simulink model "pendulum_sim"  (Simulink 7.7)
settings: Solver=ode45  StartTime=0.0  StopTime=100  RelTol=1e-3
values from neighbouring files (symbols this model uses):
  kd_th = -2*zeta_th*wn_th*AP.m2*AP.ell    [param.m]
  kd_z = AP.m2/AP.m1/AP.g*(-AP.b/AP.m2 + 2*zeta_z*wn_z)    [param.m]
  kp_th = -AP.F_max/A_th    [param.m]
  kp_z = A_th/A_z    (= 0.0174532925199)    [param.m]
undefined symbols (not defined in the file or in its folder): drawPendulum
settings Model: Creator=beard  LastModifiedBy=beard
settings OptimizationCC: InitFltsAndDblsToZero=on
settings DebuggingCC: StrictBusMsg=Warning

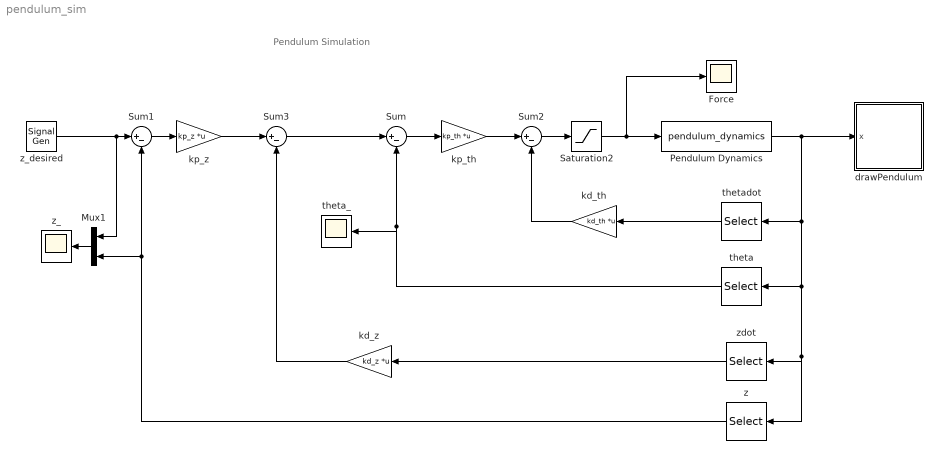
== system pendulum_sim ==
  note: Pendulum Simulation
  Force : Scope
      settings: TimeRange=100  YMin=-6  YMax=10
  Mux1 : Mux  Inputs=2
  Pendulum Dynamics : S-Function  FunctionName=pendulum_dynamics  Parameters=AP  EnableBusSupport=off
  Saturation2 : Saturate  UpperLimit=5  LowerLimit=-5
  Sum{,1..3} (4 alike) : Sum  Inputs=|+-
  drawPendulum : Subsystem
      mask init:
      | % drawing parameters
      | L = 1;
      | gap = 0.01;
      | width = 1.0;
      | height = 0.1;
      mask Display: image(imread('tv.jpg'))
  kd_th : Gain  Gain=kd_th  Multiplication=Matrix(K*u)
  kd_z : Gain  Gain=kd_z  Multiplication=Matrix(K*u)
  kp_th : Gain  Gain=kp_th  Multiplication=Matrix(K*u)
  kp_z : Gain  Gain=kp_z  Multiplication=Matrix(K*u)
  theta : Selector  InputPortWidth=4  IndexOptions=Index vector (dialog)  Indices=[2]  OutputSizes=1
  theta_ : Scope
      settings: TimeRange=100  YMin=-0.2  YMax=0.2
  thetadot : Selector  InputPortWidth=4  IndexOptions=Index vector (dialog)  Indices=[4]  OutputSizes=1
  z : Selector  InputPortWidth=4  IndexOptions=Index vector (dialog)  Indices=[1]  OutputSizes=1
  z_ : Scope
      settings: TimeRange=100  YMin=-2  YMax=2  SaveName=ScopeData2
  z_desired : SignalGenerator  WaveForm=square  Frequency=.02
  zdot : Selector  InputPortWidth=4  IndexOptions=Index vector (dialog)  Indices=[3]  OutputSizes=1
  wires:
  Pendulum Dynamics/1 -> drawPendulum/1(x), theta/1, z/1, zdot/1, thetadot/1
  Sum2/1 -> Saturation2/1
  Sum/1 -> kp_th/1
  theta/1 -> Sum/2, theta_/1
  z/1 -> Sum1/2, Mux1/2
  z_desired/1 -> Sum1/1, Mux1/1
  Mux1/1 -> z_/1
  thetadot/1 -> kd_th/1
  Sum1/1 -> kp_z/1
  kp_z/1 -> Sum3/1
  zdot/1 -> kd_z/1
  kd_z/1 -> Sum3/2
  Sum3/1 -> Sum/1
  kd_th/1 -> Sum2/2
  kp_th/1 -> Sum2/1
  Saturation2/1 -> Pendulum Dynamics/1, Force/1

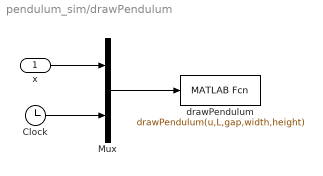
== system pendulum_sim/drawPendulum ==
  x : Inport
  Clock : Clock
      settings: Decimation=10
  Mux : Mux  Inputs=2
  drawPendulum : MATLABFcn  MATLABFcn=drawPendulum(u,L,gap,width,height)  OutputDimensions=0  SampleTime=0.1
  wires:
  Mux/1 -> drawPendulum/1
  x/1 -> Mux/1
  Clock/1 -> Mux/2
